simulink model "ButtonAndLeds_Interrupt"  (R2013b)
settings: Solver=FixedStepDiscrete  StartTime=0.0  StopTime=10.0  FixedStep=0.02  RelTol=1e-3
libraries: GPIO_Lib x3, IT_Lib x1
settings Model: Creator=reynaudp  LastModifiedBy=reynaudp
settings OptimizationCC: ExpressionDepthLimit=2147483647  OptimizeModelRefInitCode=on  LifeSpan=1
settings DebuggingCC: StateNameClashWarn=warning
settings HardwareCC: ProdLargestAtomicInteger=Integer  ProdLargestAtomicFloat=Float  ProdIntDivRoundTo=Zero  ProdEndianess=LittleEndian  ProdHWDeviceType=STMicroelectronics->STM32F4xx 32-bit Cortex-M4
settings RTWCC: SystemTargetFile=stm32F4xx.tlc  TemplateMakefile=stm32F4xx.tmf  Description=stm32F4xx (Embedded Target)  GenerateReport=on  ProcessScript=stm32F4xx_make_rtw_hook  LaunchReport=on
settings CodeAppCC: IgnoreCustomStorageClasses=off  MaxIdLength=64  CustomSymbolStrType=$N$R$M  InternalIdentifier=Classic
settings STFCustomTargetCC: ParMdlRefBuildCompliant=on  IncludeMdlTerminateFcn=off  CombineOutputUpdateFcns=on  ERTCustomFileBanners=on  SupportContinuousTime=off  SupportNonInlinedSFcns=off  MATLABClassNameForMDSCustomization=Simulink.SoftwareTarget.ERTCustomization  GRTInterface=off  SystemTargetFile=stm32F4xx.tlc
settings ERTTargetCC: CodeReplacementLibrary=ANSI_C  CompOptLevelCompliant=off  ConcurrentExecutionCompliant=off  IncludeMdlTerminateFcn=off  ERTFirstTimeCompliant=off  ModelStepFunctionPrototypeControlCompliant=off  CPPClassGenCompliant=off  InlinedParameterPlacement=NonHierarchical  ERTSrcFileBannerTemplate=sourceFileTemplate.cgt  ERTHdrFileBannerTemplate=sourceFileTemplate.cgt  ERTDataSrcFileTemplate=sourceFileTemplate.cgt  ERTDataHdrFileTemplate=sourceFileTemplate.cgt  ERTCustomFileTemplate=customRoutineProcess.tlc

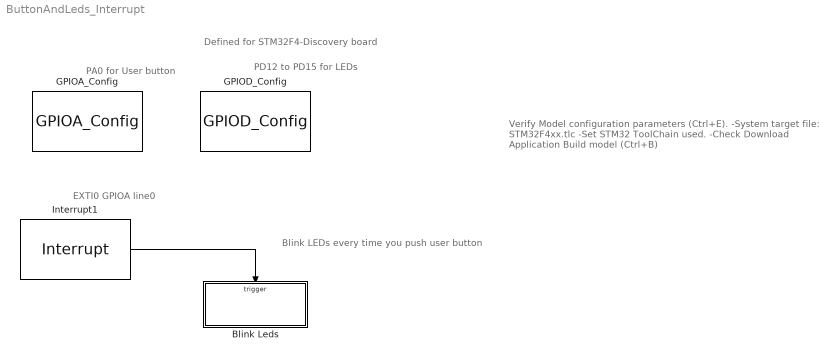
== system ButtonAndLeds_Interrupt ==
  note: Verify Model configuration parameters (Ctrl+E).
      | 	-System target file: STM32F4xx.tlc
      | 	-Set STM32 ToolChain used.
      | 	-Check Download Application
      | Build model (Ctrl+B)
  note: Blink LEDs every time you push user button
  note: EXTI0 GPIOA line0
  note: Defined for STM32F4-Discovery board
  note: PD12 to PD15 for LEDs
  note: PA0 for User button
  Blink Leds : Subsystem  TreatAsAtomicUnit=on
  GPIOA_Config : GPIO_Lib/GPIOA_Config  Pin0_Use=on  Pin1_Use=off  Pin2_Use=off  Pin3_Use=off  Pin4_Use=off  Pin5_Use=off  Pin6_Use=off  Pin7_Use=off  Pin8_Use=off  Pin9_Use=off  Pin10_Use=off  Pin11_Use=off  Pin12_Use=off  Pin13_Use=off  Pin14_Use=off  Pin15_Use=off  Pin0_Speed=GPIO_Speed_50MHz  Pin1_Speed=GPIO_Speed_2MHz  Pin2_Speed=GPIO_Speed_2MHz  Pin3_Speed=GPIO_Speed_2MHz  Pin4_Speed=GPIO_Speed_2MHz  Pin5_Speed=GPIO_Speed_2MHz  Pin6_Speed=GPIO_Speed_2MHz  Pin7_Speed=GPIO_Speed_2MHz  Pin8_Speed=GPIO_Speed_2MHz  Pin9_Speed=GPIO_Speed_2MHz  Pin10_Speed=GPIO_Speed_2MHz  Pin11_Speed=GPIO_Speed_2MHz  Pin12_Speed=GPIO_Speed_2MHz  Pin13_Speed=GPIO_Speed_2MHz  Pin14_Speed=GPIO_Speed_2MHz  Pin15_Speed=GPIO_Speed_2MHz  Pin0_Mode=GPIO_Mode_IN  Pin1_Mode=GPIO_Mode_OUT  Pin2_Mode=GPIO_Mode_OUT  Pin3_Mode=GPIO_Mode_OUT  Pin4_Mode=GPIO_Mode_OUT  Pin5_Mode=GPIO_Mode_OUT  Pin6_Mode=GPIO_Mode_OUT  Pin7_Mode=GPIO_Mode_OUT  Pin8_Mode=GPIO_Mode_OUT  Pin9_Mode=GPIO_Mode_OUT  Pin10_Mode=GPIO_Mode_OUT  Pin11_Mode=GPIO_Mode_OUT  Pin12_Mode=GPIO_Mode_OUT  Pin13_Mode=GPIO_Mode_OUT  Pin14_Mode=GPIO_Mode_OUT  Pin15_Mode=GPIO_Mode_OUT  Pin0_Type=GPIO_OType_PP  Pin1_Type=GPIO_OType_PP  Pin2_Type=GPIO_OType_PP  Pin3_Type=GPIO_OType_PP  Pin4_Type=GPIO_OType_PP  Pin5_Type=GPIO_OType_PP  Pin6_Type=GPIO_OType_PP  Pin7_Type=GPIO_OType_PP  Pin8_Type=GPIO_OType_PP  Pin9_Type=GPIO_OType_PP  Pin10_Type=GPIO_OType_PP  Pin11_Type=GPIO_OType_PP  Pin12_Type=GPIO_OType_PP  Pin13_Type=GPIO_OType_PP  Pin14_Type=GPIO_OType_PP  Pin15_Type=GPIO_OType_PP  Pin0_PuPd=GPIO_PuPd_NOPULL  Pin1_PuPd=GPIO_PuPd_NOPULL  Pin2_PuPd=GPIO_PuPd_NOPULL  Pin3_PuPd=GPIO_PuPd_NOPULL  Pin4_PuPd=GPIO_PuPd_NOPULL  Pin5_PuPd=GPIO_PuPd_NOPULL  Pin6_PuPd=GPIO_PuPd_NOPULL  Pin7_PuPd=GPIO_PuPd_NOPULL  Pin8_PuPd=GPIO_PuPd_NOPULL  Pin9_PuPd=GPIO_PuPd_NOPULL  Pin10_PuPd=GPIO_PuPd_NOPULL  Pin11_PuPd=GPIO_PuPd_NOPULL  Pin12_PuPd=GPIO_PuPd_NOPULL  Pin13_PuPd=GPIO_PuPd_NOPULL  Pin14_PuPd=GPIO_PuPd_NOPULL  Pin15_PuPd=GPIO_PuPd_NOPULL  Pin0_AF=GPIO_AF_TIM2  Pin1_AF=GPIO_AF_TIM2  Pin2_AF=GPIO_AF_TIM2  Pin3_AF=GPIO_AF_TIM2  Pin4_AF=GPIO_AF_SPI1  Pin5_AF=GPIO_AF_EVENTOUT  Pin6_AF=GPIO_AF_TIM1  Pin7_AF=GPIO_AF_TIM1  Pin8_AF=GPIO_AF_MCO  Pin9_AF=GPIO_AF_TIM1  Pin10_AF=GPIO_AF_TIM1  Pin11_AF=GPIO_AF_TIM1  Pin12_AF=GPIO_AF_TIM1  Pin13_AF=GPIO_AF_SWJ  Pin14_AF=GPIO_AF_SWJ  Pin15_AF=GPIO_AF_EVENTOUT  Pin0_Set=off  Pin1_Set=off  Pin2_Set=off  Pin3_Set=off  Pin4_Set=off  Pin5_Set=off  Pin6_Set=off  Pin7_Set=off  Pin8_Set=off  Pin9_Set=off  Pin10_Set=off  Pin11_Set=off  Pin12_Set=off  Pin13_Set=off  Pin14_Set=off  Pin15_Set=off
  GPIOD_Config : GPIO_Lib/GPIOD_Config  Pin0_Use=off  Pin1_Use=off  Pin2_Use=off  Pin3_Use=off  Pin4_Use=off  Pin5_Use=off  Pin6_Use=off  Pin7_Use=off  Pin8_Use=off  Pin9_Use=off  Pin10_Use=off  Pin11_Use=off  Pin12_Use=on  Pin13_Use=on  Pin14_Use=on  Pin15_Use=on  Pin0_Speed=GPIO_Speed_2MHz  Pin1_Speed=GPIO_Speed_2MHz  Pin2_Speed=GPIO_Speed_2MHz  Pin3_Speed=GPIO_Speed_2MHz  Pin4_Speed=GPIO_Speed_2MHz  Pin5_Speed=GPIO_Speed_2MHz  Pin6_Speed=GPIO_Speed_2MHz  Pin7_Speed=GPIO_Speed_2MHz  Pin8_Speed=GPIO_Speed_2MHz  Pin9_Speed=GPIO_Speed_2MHz  Pin10_Speed=GPIO_Speed_2MHz  Pin11_Speed=GPIO_Speed_2MHz  Pin12_Speed=GPIO_Speed_50MHz  Pin13_Speed=GPIO_Speed_50MHz  Pin14_Speed=GPIO_Speed_50MHz  Pin15_Speed=GPIO_Speed_50MHz  Pin0_Mode=GPIO_Mode_OUT  Pin1_Mode=GPIO_Mode_OUT  Pin2_Mode=GPIO_Mode_OUT  Pin3_Mode=GPIO_Mode_OUT  Pin4_Mode=GPIO_Mode_OUT  Pin5_Mode=GPIO_Mode_OUT  Pin6_Mode=GPIO_Mode_OUT  Pin7_Mode=GPIO_Mode_OUT  Pin8_Mode=GPIO_Mode_OUT  Pin9_Mode=GPIO_Mode_OUT  Pin10_Mode=GPIO_Mode_OUT  Pin11_Mode=GPIO_Mode_OUT  Pin12_Mode=GPIO_Mode_OUT  Pin13_Mode=GPIO_Mode_OUT  Pin14_Mode=GPIO_Mode_OUT  Pin15_Mode=GPIO_Mode_OUT  Pin0_Type=GPIO_OType_PP  Pin1_Type=GPIO_OType_PP  Pin2_Type=GPIO_OType_PP  Pin3_Type=GPIO_OType_PP  Pin4_Type=GPIO_OType_PP  Pin5_Type=GPIO_OType_PP  Pin6_Type=GPIO_OType_PP  Pin7_Type=GPIO_OType_PP  Pin8_Type=GPIO_OType_PP  Pin9_Type=GPIO_OType_PP  Pin10_Type=GPIO_OType_PP  Pin11_Type=GPIO_OType_PP  Pin12_Type=GPIO_OType_PP  Pin13_Type=GPIO_OType_PP  Pin14_Type=GPIO_OType_PP  Pin15_Type=GPIO_OType_PP  Pin0_PuPd=GPIO_PuPd_NOPULL  Pin1_PuPd=GPIO_PuPd_NOPULL  Pin2_PuPd=GPIO_PuPd_NOPULL  Pin3_PuPd=GPIO_PuPd_NOPULL  Pin4_PuPd=GPIO_PuPd_NOPULL  Pin5_PuPd=GPIO_PuPd_NOPULL  Pin6_PuPd=GPIO_PuPd_NOPULL  Pin7_PuPd=GPIO_PuPd_NOPULL  Pin8_PuPd=GPIO_PuPd_NOPULL  Pin9_PuPd=GPIO_PuPd_NOPULL  Pin10_PuPd=GPIO_PuPd_NOPULL  Pin11_PuPd=GPIO_PuPd_NOPULL  Pin12_PuPd=GPIO_PuPd_NOPULL  Pin13_PuPd=GPIO_PuPd_NOPULL  Pin14_PuPd=GPIO_PuPd_NOPULL  Pin15_PuPd=GPIO_PuPd_NOPULL  Pin0_AF=GPIO_AF_CAN1  Pin1_AF=GPIO_AF_CAN1  Pin2_AF=GPIO_AF_TIM3  Pin3_AF=GPIO_AF_USART2  Pin4_AF=GPIO_AF_USART2  Pin5_AF=GPIO_AF_EVENTOUT  Pin6_AF=GPIO_AF_USART2  Pin7_AF=GPIO_AF_USART2  Pin8_AF=GPIO_AF_USART3  Pin9_AF=GPIO_AF_USART3  Pin10_AF=GPIO_AF_USART3  Pin11_AF=GPIO_AF_USART3  Pin12_AF=GPIO_AF_TIM4  Pin13_AF=GPIO_AF_TIM4  Pin14_AF=GPIO_AF_TIM4  Pin15_AF=GPIO_AF_EVENTOUT  Pin0_Set=off  Pin1_Set=off  Pin2_Set=off  Pin3_Set=off  Pin4_Set=off  Pin5_Set=off  Pin6_Set=off  Pin7_Set=off  Pin8_Set=off  Pin9_Set=off  Pin10_Set=off  Pin11_Set=off  Pin12_Set=off  Pin13_Set=off  Pin14_Set=off  Pin15_Set=off
  Interrupt1 : IT_Lib/Interrupt  Peripheral_name=EXTint  Peripheral_IRQid=11  Enable_sim=off  ADC1_en=on  ADC2_en=off  ADC3_en=off  ADC_EOC=off  ADC_JEOC=off  ADC_AWD=on  ADC_OVR=off  EXTI_port=GPIOA  EXTI_line=0  EXTI_trig=Rising  Def_handler=on  Cust_handler=EXTI0_IRQHandler  Group_prio=NVIC_PriorityGroup_0  Pre0_prio=0  Sub0_prio=0  Pre1_prio=0  Sub1_prio=0  Pre2_prio=0  Sub2_prio=0  Pre3_prio=0  Sub3_prio=0  Pre4_prio=0  Sub4_prio=0  Time_base=0.1
  wires:
  Interrupt1/1 -> Blink Leds/Trigger

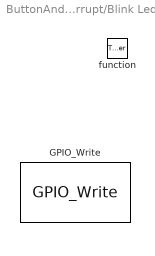
== system ButtonAndLeds_Interrupt/Blink Leds ==
  function : TriggerPort  TriggerType=function-call
  GPIO_Write : GPIO_Lib/GPIO_Write  Port_name=GPIOD  Enable_input=off  Pin0=off  Toggle_Pin0=off  Pin1=off  Toggle_Pin1=off  Pin2=off  Toggle_Pin2=off  Pin3=off  Toggle_Pin3=off  Pin4=off  Toggle_Pin4=off  Pin5=off  Toggle_Pin5=off  Pin6=off  Toggle_Pin6=off  Pin7=off  Toggle_Pin7=off  Pin8=off  Toggle_Pin8=off  Pin9=off  Toggle_Pin9=off  Pin10=off  Toggle_Pin10=off  Pin11=off  Toggle_Pin11=off  Pin12=on  Toggle_Pin12=on  Pin13=on  Toggle_Pin13=on  Pin14=on  Toggle_Pin14=on  Pin15=on  Toggle_Pin15=on
